simulink model "Suspension7DoF_GDP_Final"  (R2025a)
settings: Solver=ode4  StartTime=0.0  StopTime=209.85  FixedStep=0.001  RelTol=1e-3
undefined symbols (not defined in the file): A, Bl, Cl_table, cmax_f, cmax_r, cmax_roll_f, cmax_roll_r, cmin_f, cmin_r, cmin_roll_f, cmin_roll_r, cog_z, cog_z_us, CoP_x_table, CoP_y, g, Ixx, Iyy, k_roll_f, k_roll_r, kf, kr, kt, Lf, Lr, m_s, m_s_a, m_s_b, m_us, rake_breaks, RC_F_z, RC_R_z, RH_breaks, rho, roll_centre_z, Tr
libraries: simulink x2
settings Model: Creator=alexw  LastModifiedBy=alexw

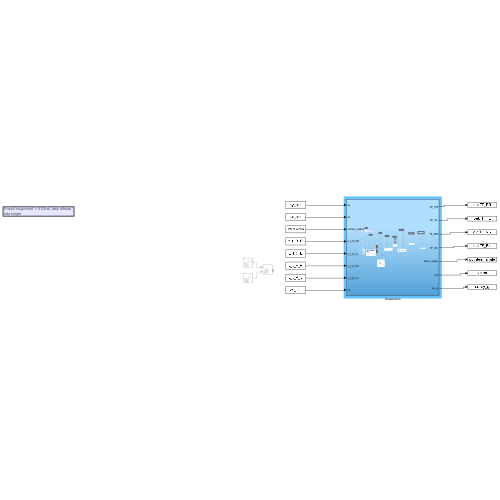
[thumbnail: Simulink's stored preview of the top-level diagram]
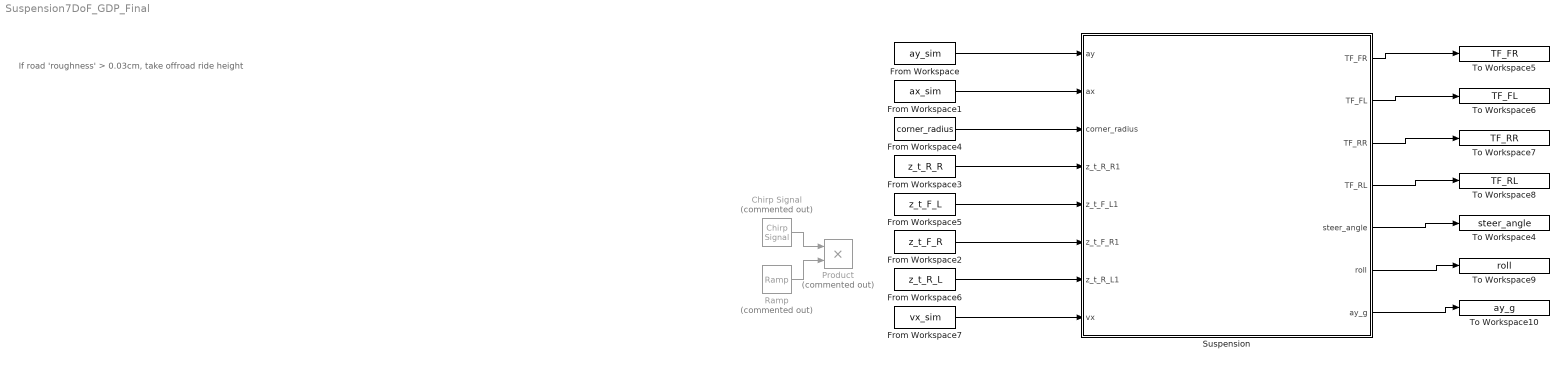
== system Suspension7DoF_GDP_Final ==
  note: If road 'roughness' > 0.03cm, take offroad
      | ride height
  Chirp Signal : simulink/Sources/Chirp Signal  Commented=on  f1=0.1  T=100  f2=20
  From Workspace : FromWorkspace  VariableName=ay_sim
  From Workspace1 : FromWorkspace  VariableName=ax_sim
  From Workspace2 : FromWorkspace  VariableName=z_t_F_R
  From Workspace3 : FromWorkspace  VariableName=z_t_R_R
  From Workspace4 : FromWorkspace  VariableName=corner_radius
  From Workspace5 : FromWorkspace  VariableName=z_t_F_L
  From Workspace6 : FromWorkspace  VariableName=z_t_R_L
  From Workspace7 : FromWorkspace  VariableName=vx_sim
  Product : Product  Commented=on
  Ramp : simulink/Sources/Ramp  Commented=on  slope=-0.0001  start=0  InitialOutput=0.01
  Suspension : Subsystem
  To Workspace10 : ToWorkspace  VariableName=ay_g  SaveFormat=Timeseries  SampleTime=-1
  To Workspace4 : ToWorkspace  VariableName=steer_angle  SaveFormat=Timeseries  SampleTime=-1
  To Workspace5 : ToWorkspace  VariableName=TF_FR  SaveFormat=Timeseries  SampleTime=-1
  To Workspace6 : ToWorkspace  VariableName=TF_FL  SaveFormat=Timeseries  SampleTime=-1
  To Workspace7 : ToWorkspace  VariableName=TF_RR  SaveFormat=Timeseries  SampleTime=-1
  To Workspace8 : ToWorkspace  VariableName=TF_RL  SaveFormat=Timeseries  SampleTime=-1
  To Workspace9 : ToWorkspace  VariableName=roll  SaveFormat=Timeseries  SampleTime=-1
  wires:
  Chirp Signal/1 -> Product/1
  Ramp/1 -> Product/2
  From Workspace/1 -> Suspension/1(ay)
  From Workspace1/1 -> Suspension/2(ax)
  From Workspace3/1 -> Suspension/4(z_t_R_R1)
  Suspension/1(TF_FR) -> To Workspace5/1
  Suspension/2(TF_FL) -> To Workspace6/1
  Suspension/3(TF_RR) -> To Workspace7/1
  Suspension/4(TF_RL) -> To Workspace8/1
  Suspension/5(steer_angle) -> To Workspace4/1
  From Workspace4/1 -> Suspension/3(corner_radius)
  From Workspace5/1 -> Suspension/5(z_t_F_L1)
  Suspension/6(roll) -> To Workspace9/1
  Suspension/7(ay_g) -> To Workspace10/1
  From Workspace7/1 -> Suspension/8(vx)
  From Workspace6/1 -> Suspension/7(z_t_R_L1)
  From Workspace2/1 -> Suspension/6(z_t_F_R1)

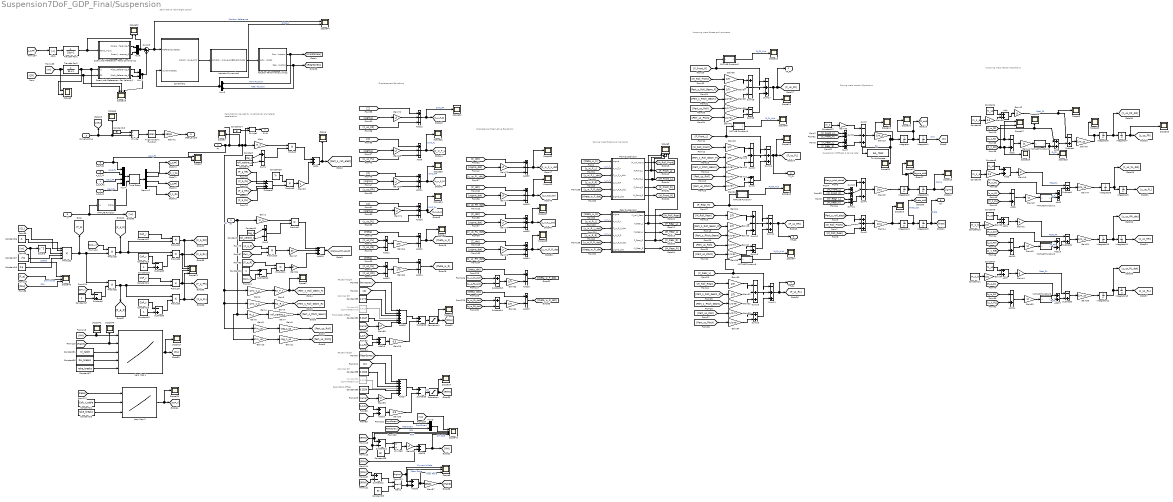
== system Suspension7DoF_GDP_Final/Suspension ==
  note: Suspension Stiffness = spring rate:
  note: Unsprung mass Newton Equations
  note: Sprung mass newton Equations
  note: Unsprung mass forces and moments
  note: Sprung mass forces and moments
  note: Displacement Derivative Equations
  note: Displacement Equations
  note: Perturbations caused by
      | longitudinal and lateral acceleration
  note: Front Static Offset
  note: Rear Static Offset
  note: Raised height
  note: Raised height
  note: Nominal RH
  note: Nominal RH
  note: Semi-Active ride height control
  ay : Inport
  ax : Inport  Port=2
  corner_radius : Inport  Port=3
  z_t_R_R1 : Inport  Port=4
  z_t_F_L1 : Inport  Port=5
  z_t_F_R1 : Inport  Port=6
  z_t_R_L1 : Inport  Port=7
  vx : Inport  Port=8
  Abs1 : Abs  SaturateOnIntegerOverflow=off
  Actuator Dynamics1 : Subsystem
  Actuator Performance Limits1 : Subsystem
  Add{,1,3..5,7,9,13,17,19..20,28,30} (13 alike) : Sum
  Add{2,6,10,14} (4 alike) : Sum  Inputs=-+
  Add{11,16,34..35} (4 alike) : Sum  Inputs=++-
  Add{8,12,15,33} (4 alike) : Sum  Inputs=+--
  Add18 : Sum  Inputs=+++
  Add{21..25,29} (6 alike) : Sum  Inputs=+-
  Add26 : Sum  Inputs=++++++
  Add27 : Sum  Inputs=++++++
  Aero Map 1 : Lookup_n-D  LookupTableObject=h  BreakpointsForDimension1Source=Input port  BreakpointsForDimension1=[0:0.01:0.2]  BreakpointsForDimension2Source=Input port  BreakpointsForDimension2=[-10:10]  TableSource=Input port  InternalRulePriority=Speed  RndMeth=Simplest
      settings: InputPortMap=u0,u1,p221,p5,p7
  Aero Map 2 : Lookup_n-D  NumberOfTableDimensions=1  BreakpointsForDimension1Source=Input port  BreakpointsForDimension1=[-5:5]  TableSource=Input port  Table=tanh([-5:5])  InternalRulePriority=Speed  RndMeth=Simplest
      settings: InputPortMap=u0,p221,p5
  Atan2 : Trigonometry  Operator=atan2
  Constant : Constant  Value=cog_z
  Constant1 : Constant  Value=roll_centre_z
  Constant10 : Constant  Value=m_s_b
  Constant11 : Constant  Value=m_s_b
  Constant12 : Constant  Value=m_s
  Constant13 : Constant  Value=Bl
  Constant14 : Constant  Value=g
  Constant15 : Constant  Commented=on  Value=0.025
  Constant16 : Constant  Value=0.5
  Constant{17..20} (4 alike) : Constant
  Constant2 : Constant  Value=cog_z
  Constant21 : Constant  Value=CoP_x_table  VectorParams1D=off
  Constant{22..25} (4 alike) : Constant  Value=CoP_y
  Constant26 : Constant  Value=A
  Constant27 : Constant  Value=rho
  Constant28 : Constant  Value=Tr
  Constant29 : Constant  Value=rake_breaks  VectorParams1D=off
  Constant3 : Constant  Value=roll_centre_z
  Constant30 : Constant  Value=0.1154
  Constant31 : Constant  Value=Cl_table  VectorParams1D=off
  Constant32 : Constant  Value=0.1447
  Constant33 : Constant  Value=Bl
  Constant34 : Constant  Commented=on  Value=0.025
  Constant35 : Constant  Value=0.1043
  Constant36 : Constant  Value=RH_breaks  VectorParams1D=off
  Constant37 : Constant  Value=rake_breaks  VectorParams1D=off
  Constant38 : Constant  Value=Bl
  Constant39 : Constant  Value=0.075
  Constant{4..7} (4 alike) : Constant  Value=m_us
  Constant8 : Constant  Value=m_s_a
  Constant9 : Constant  Value=m_s_a
  Controller1 : Subsystem
  Demux1 : Demux
  Divide : Product  Inputs=*/
  Divide1 : Product  Inputs=*/
  Divide3 : Product  Inputs=*/
  Front Suspension : Subsystem  mask(half-car suspension){kf=kf, kthetaf=-k_roll_f, cmin_f=cmin_f, cmax_f=cmax_f, cmin_thetaf=cmin_roll_f, cmax_thetaf=cmax_roll_f, Lr=Lr}
      mask prompts: kf "Suspension Stiffness"; kthetaf "Roll Stiffness:"; cmin_f "Minmum Suspension Damping:"; cmax_f "Maximum Suspension Damping:"; cmin_thetaf "Minimum Roll Damping:"; cmax_thetaf "Maximum Roll Damping:"; Lr "Moment Arm:"
      mask help:
      | Half-Car Suspension
      | The spring and damping rates for an individual wheel are entered below.  Their combined effect as applied to two wheels at the specified distance from the center of mass is computed.  The distance should be specified as positive if the subsystem is oriented such that increasing z corresponds to increasing theta, negative otherwise.
      mask Help: See "Using Simulink and Stateflow in Automotive Applications" for a mathematical derivation of the subsystem operation.  Contact your MathWorks distributor to obtain a copy.
      mask Display: plot(-1, 0, 13, 12, [1 12], [11 11], [1 5], [2 2], [1 2], [4.5 5], [2 0], [5 6], [0 2], [6 7], [2 0], [7 8], [0 1], [8 8.5], [1 1], [8.5 11], [1 1], [2 4.5], [5 5], [2 5], [4 6], [5 5], [4 4], [5 8], [6 6], [5 8], [4 6], [6.5 6.5], [5 5], [6.5 11], [0 1], [1 2], [2 3], [1 2], [4 5], [1 2])
  Gain : Gain  Gain=m_s
  Gain1 : Gain  Gain=m_s
  Gain10 : Gain  Gain=4*m_us
  Gain11 : Gain  Gain=cog_z_us
  Gain{12,16,42,44,46} (5 alike) : Gain  Gain=g
  Gain13 : Gain  Gain=1/m_s
  Gain14 : Gain  Gain=1/Ixx
  Gain15 : Gain  Gain=1/Iyy
  Gain17 : Gain  Gain=Bl
  Gain{18..19,24..25,30..31,36..37,60..62,64} (12 alike) : Gain  Gain=1/Tr
  Gain2 : Gain  Gain=-1*m_s_a
  Gain{20,22,26,28,32,34,38,40} (8 alike) : Gain  Gain=1/(2*Bl)
  Gain{21,27,33,39} (4 alike) : Gain  Gain=1/(2*Tr)
  Gain23 : Gain
  Gain{29,35,48,50,52,54} (6 alike) : Gain  Gain=0.5
  Gain3 : Gain  Gain=RC_F_z
  Gain4 : Gain  Gain=-1*m_s_b
  Gain{41,45,49,53} (4 alike) : Gain  Gain=kt
  Gain{43,47,51,55} (4 alike) : Gain  Gain=1/m_us
  Gain5 : Gain  Gain=RC_R_z
  Gain56 : Gain  Gain=Bl
  Gain57 : Gain  Gain=180/pi
  Gain{58,63,68,70,73..74} (6 alike) : Gain  Gain=Lf
  Gain59 : Gain  Gain=-Lr
  Gain6 : Gain  Gain=m_s
  Gain{69,71,75..76} (4 alike) : Gain  Gain=Lr
  Gain7 : Gain  Gain=roll_centre_z
  Gain72 : Gain  Gain=180/pi
  Gain8 : Gain  Gain=4*m_us
  Gain9 : Gain  Gain=cog_z_us
  Integrator{,1..13} (14 alike) : Integrator
  MATLAB Function : MATLAB Function  TreatAsAtomicUnit=on
  MATLAB Function1 : MATLAB Function  TreatAsAtomicUnit=on
  MATLAB Function2 : MATLAB Function  TreatAsAtomicUnit=on
  MATLAB Function3 : MATLAB Function  TreatAsAtomicUnit=on
  MATLAB Function4 : MATLAB Function  TreatAsAtomicUnit=on
  MATLAB Function5 : MATLAB Function  TreatAsAtomicUnit=on
  MATLAB Function6 : MATLAB Function  TreatAsAtomicUnit=on
  MATLAB Function7 : MATLAB Function  TreatAsAtomicUnit=on
  MATLAB Function8 : MATLAB Function  TreatAsAtomicUnit=on
  Mux{3,5..7} (4 alike) : Mux  Inputs=2
  Mux4 : Mux
  Product{,1,3..11} (11 alike) : Product
  Product2 : Product  Inputs=5
  Rear Suspension : Subsystem  mask(half-car suspension){kr=kr, kthetar=-k_roll_r, cmin_r=cmin_r, cmax_r=cmax_r, cmin_thetar=cmin_roll_r, cmax_thetar=cmax_roll_r, Lr=Lr}
      mask prompts: kr "Suspension Stiffness:"; kthetar "Roll Stiffness:"; cmin_r "Minimum Suspension Damping:"; cmax_r "Maximum Suspension Damping:"; cmin_thetar "Minimum Roll Damping:"; cmax_thetar "Maximum Roll Damping:"; Lr "Moment Arm:"
      mask help:
      | Half-Car Suspension
      | The spring and damping rates for an individual wheel are entered below.  Their combined effect as applied to two wheels at the specified distance from the center of mass is computed.  The distance should be specified as positive if the subsystem is oriented such that increasing z corresponds to increasing theta, negative otherwise.
      mask Help: See "Using Simulink and Stateflow in Automotive Applications" for a mathematical derivation of the subsystem operation.  Contact your MathWorks distributor to obtain a copy.
      mask Display: plot(-1, 0, 13, 12, [1 12], [11 11], [1 5], [2 2], [1 2], [4.5 5], [2 0], [5 6], [0 2], [6 7], [2 0], [7 8], [0 1], [8 8.5], [1 1], [8.5 11], [1 1], [2 4.5], [5 5], [2 5], [4 6], [5 5], [4 4], [5 8], [6 6], [5 8], [4 6], [6.5 6.5], [5 5], [6.5 11], [0 1], [1 2], [2 3], [1 2], [4 5], [1 2])
  Saturation : Saturate  LowerLimit=0
  Saturation1 : Saturate  LowerLimit=0
  Scope{,1..4,6,10..15,17..20,23..26,28..39,42..43,45..47} (37 alike) : Scope
      Scope settings: DataLoggingVariableName=ScopeData28
      Scope1 settings: ActiveDisplayYMinimum=-15.845612610428327  ActiveDisplayYMaximum=15.435881700857845  DataLoggingVariableName=ScopeData13
      Scope10 settings: ActiveDisplayYMinimum=-1  ActiveDisplayYMaximum=1  DataLoggingVariableName=ScopeData14
      Scope11 settings: ActiveDisplayYMinimum=-1  ActiveDisplayYMaximum=1  DataLoggingVariableName=ScopeData15
      Scope12 settings: ActiveDisplayYMinimum=-1  ActiveDisplayYMaximum=1  DataLoggingVariableName=ScopeData16
      Scope13 settings: ActiveDisplayYMinimum=-0.11164438440318229  ActiveDisplayYMaximum=0.015517013432769977  DataLoggingVariableName=ScopeData17
      Scope14 settings: ActiveDisplayYMinimum=-1  ActiveDisplayYMaximum=1  DataLoggingVariableName=ScopeData18
      Scope15 settings: DataLoggingVariableName=ScopeData19
      Scope17 settings: ActiveDisplayYMinimum=-1.4006676134136735  ActiveDisplayYMaximum=0.60935482779584749  DataLoggingVariableName=ScopeData35
      Scope18 settings: DataLoggingVariableName=ScopeData22
      Scope19 settings: ActiveDisplayYMinimum=-1  ActiveDisplayYMaximum=1  DataLoggingVariableName=ScopeData23
      Scope2 settings: ActiveDisplayYMinimum=-1  ActiveDisplayYMaximum=1  DataLoggingVariableName=ScopeData6
      Scope20 settings: ActiveDisplayYMinimum=-1  ActiveDisplayYMaximum=1  DataLoggingVariableName=ScopeData24
      Scope23 settings: ActiveDisplayYMinimum=-1  ActiveDisplayYMaximum=1  DataLoggingVariableName=ScopeData36
      Scope24 settings: ActiveDisplayYMinimum=-1  ActiveDisplayYMaximum=1  DataLoggingVariableName=ScopeData37
      Scope25 settings: ActiveDisplayYMinimum=-2095.00512229594  ActiveDisplayYMaximum=18855.046100663465  DataLoggingVariableName=ScopeData29
      Scope26 settings: ActiveDisplayYMinimum=-0.15055367778646628  ActiveDisplayYMaximum=0.064777386245955387  DataLoggingVariableName=ScopeData30
      Scope28 settings: ActiveDisplayYMinimum=-0.00037040753132380039  ActiveDisplayYMaximum=0.0017989620179888006  DataLoggingVariableName=ScopeData32
      Scope29 settings: ActiveDisplayYMinimum=-14729.679405263418  ActiveDisplayYMaximum=5136.5247908965184  DataLoggingVariableName=ScopeData33
      Scope3 settings: ActiveDisplayYMinimum=-1  ActiveDisplayYMaximum=1  DataLoggingVariableName=ScopeData7
      Scope30 settings: ActiveDisplayYMinimum=-1  ActiveDisplayYMaximum=1  DataLoggingVariableName=ScopeData34
      Scope31 settings: ActiveDisplayYMinimum=-0.35226875587213935  ActiveDisplayYMaximum=0.075007941544787432  DataLoggingVariableName=ScopeData6
      Scope32 settings: ActiveDisplayYMinimum=-0.26331111069166768  ActiveDisplayYMaximum=0.0678002738486741  DataLoggingVariableName=ScopeData29
      Scope33 settings: ActiveDisplayYMinimum=-0.28108589618879348  ActiveDisplayYMaximum=0.05450271554919274  DataLoggingVariableName=ScopeData4
      Scope34 settings: ActiveDisplayYMinimum=-0.024162682451583074  ActiveDisplayYMaximum=0.024369090839316668  DataLoggingVariableName=ScopeData5
      Scope35 settings: ActiveDisplayYMinimum=-1.8920079045633775  ActiveDisplayYMaximum=1.5269548555882952
      Scope36 settings: ActiveDisplayYMinimum=-1.8920079045633775  ActiveDisplayYMaximum=1.5269548555882952
      Scope37 settings: ActiveDisplayYMinimum=-2.8014124962622828  ActiveDisplayYMaximum=2.3840420433740279  DataLoggingVariableName=ScopeData2
      Scope38 settings: ActiveDisplayYMinimum=-2.8014124962622828  ActiveDisplayYMaximum=2.3840420433740279  DataLoggingVariableName=ScopeData3
      Scope39 settings: ActiveDisplayYMinimum=-1  ActiveDisplayYMaximum=1  DataLoggingVariableName=ScopeData38
      Scope4 settings: ActiveDisplayYMinimum=-1  ActiveDisplayYMaximum=1  DataLoggingVariableName=ScopeData8
      Scope42 settings: ActiveDisplayYMinimum=-1  ActiveDisplayYMaximum=1  DataLoggingVariableName=ScopeData41
      Scope43 settings: ActiveDisplayYMinimum=-9.022413114497672  ActiveDisplayYMaximum=5.2150908469293062  DataLoggingVariableName=ScopeData42
      Scope45 settings: DataLoggingVariableName=ScopeData20
      Scope46 settings: DataLoggingVariableName=ScopeData45
      Scope47 settings: DataLoggingVariableName=ScopeData46
      Scope6 settings: ActiveDisplayYMinimum=-20.40704420043474  ActiveDisplayYMaximum=1207.4194628810842  DataLoggingVariableName=ScopeData10
  Scope16 : Scope  NumInputPorts=3
      settings: ActiveDisplayString=3  ActiveDisplayYMinimum=-0.012499999999999997  ActiveDisplayYMaximum=0.1125  DataLoggingVariableName=ScopeData27
  Scope21 : Scope  NumInputPorts=4
      settings: ActiveDisplayYMinimum=-1  ActiveDisplayYMaximum=1  DataLoggingVariableName=ScopeData26
  Scope{7..8,22,27,44} (5 alike) : Scope  NumInputPorts=2
      Scope22 settings: ActiveDisplayYMinimum=-0.0093749999999999979  ActiveDisplayYMaximum=0.084374999999999992  DataLoggingVariableName=ScopeData43
      Scope27 settings: ActiveDisplayYMinimum=-1  ActiveDisplayYMaximum=1  DataLoggingVariableName=ScopeData31
      Scope44 settings: ActiveDisplayYMinimum=-0.012499999999999997  ActiveDisplayYMaximum=0.1125  DataLoggingVariableName=ScopeData44
      Scope7 settings: ActiveDisplayYMinimum=-11.512910069370855  ActiveDisplayYMaximum=11.657951350029352  DataLoggingVariableName=ScopeData11
      Scope8 settings: ActiveDisplayYMinimum=-1  ActiveDisplayYMaximum=1
  Scope40 : Scope  NumInputPorts=3
      settings: ActiveDisplayYMinimum=-1  ActiveDisplayYMaximum=1  DataLoggingVariableName=ScopeData39
  Scope41 : Scope  NumInputPorts=5
      settings: ActiveDisplayYMinimum=-6.374509016200431  ActiveDisplayYMaximum=57.4705811458039  DataLoggingVariableName=ScopeData40
  Scope5 : Scope  NumInputPorts=3
      settings: ActiveDisplayYMinimum=-1  ActiveDisplayYMaximum=1  DataLoggingVariableName=ScopeData9
  Scope9 : Scope  NumInputPorts=4
      settings: ActiveDisplayYMinimum=-1  ActiveDisplayYMaximum=1  DataLoggingVariableName=ScopeData25
  Screw jack Reference - Car Velocity1 : MATLAB Function  TreatAsAtomicUnit=on
  Screw jack Reference - Road Conditions1 : MATLAB Function  TreatAsAtomicUnit=on
  Square : Math  Operator=square
  Subtract{,1..6} (7 alike) : Sum  Inputs=-+
  Subtract{8..14} (7 alike) : Sum  Inputs=+-
  Subtract7 : Sum  Inputs=+-+-
  Sum1 : Sum  Inputs=|+-
  Sum{10..11,14..15,17} (5 alike) : Sum  Inputs=|-++
  Sum12 : Sum  Inputs=|+-+
  Sum13 : Sum  Inputs=|-+
  Sum16 : Sum  Inputs=|++
  Sum18 : Sum  Inputs=|+--
  Sum19 : Sum  Inputs=|--
  Sum2 : Sum  Inputs=|+-
  Sum{5,7,20..21} (4 alike) : Sum
  Sum23 : Sum  Inputs=|++
  Sum3 : Sum  Inputs=-++
  Sum4 : Sum  Inputs=|+-+
  Sum6 : Sum  Inputs=|+++
  Sum8 : Sum  Inputs=|-+-
  Sum9 : Sum  Inputs=|+-
  Time Delay : VariableTransportDelay  MaximumDelay=10  MaximumPoints=10240  FixedBuffer=on  ZeroDelay=on
  To Workspace : ToWorkspace  VariableName=BA_7DoF  SampleTime=-1
      settings: Save2DSignal=2-D array (concatenate along first dimension)
  Transfer Fcn1 : TransferFcn  Denominator=[10 1]
  Transfer Fcn2 : TransferFcn  Denominator=[3 1]
  Trigonometric Function : Trigonometry  Operator=atan
  TF_FR : Outport
  TF_FL : Outport  Port=2
  TF_RR : Outport  Port=3
  TF_RL : Outport  Port=4
  steer_angle : Outport  Port=5
  roll : Outport  Port=6
  ay_g : Outport  Port=7
  wires:
  Gain/1 -> Product/1
  Constant1/1 -> Sum1/2
  Constant/1 -> Sum1/1
  Sum1/1 -> Product/2
  Constant2/1 -> Sum2/1
  Constant3/1 -> Sum2/2
  Gain1/1 -> Product1/1
  ax/1 -> Gain1/1, Gain10/1, Gain6/1
  Sum2/1 -> Product1/2
  Gain2/1 -> Gain3/1
  Gain4/1 -> Gain5/1
  Gain3/1 -> Scope2/1, [Pert_s_Roll_Geom_F]
  Gain5/1 -> [Pert_s_Roll_Geom_R]
  Gain6/1 -> Gain7/1
  Gain7/1 -> [Pert_s_Pitch_Geom]
  Gain8/1 -> Gain9/1
  Gain10/1 -> Gain11/1
  Gain9/1 -> [Pert_us_Roll]
  Gain11/1 -> [Pert_us_Pitch]
  Sum3/1 -> Gain13/1
  Gain13/1 -> To Workspace/1, Scope30/1, Scope11/1, Integrator/1  "BA"
  Integrator/1 -> Scope10/1, [Z_dot], Integrator1/1
  Integrator2/1 -> Scope12/1, [sigma_dot], Integrator3/1
  Gain15/1 -> Integrator2/1
  Sum4/1 -> Gain15/1
  [Pert_s_pitch_elast] -> Sum4/1
  [Pert_s_roll_elast] -> Sum6/1
  Integrator5/1 -> roll/1, [theta]  "theta"
  Sum6/1 -> Gain14/1
  [M_Roll_Rear] -> Sum6/3
  [M_Roll_Front] -> Sum6/2
  Gain14/1 -> Scope19/1, Integrator4/1
  Sum8/1 -> Sum10/2
  Sum9/1 -> Sum10/3
  Sum10/1 -> TF_FL/1, Scope18/1, [F_us_FL]
  [M_Roll_Front] -> Gain18/1
  Gain18/1 -> Sum8/1
  [Pert_s_Roll_Geom_F] -> Gain19/1
  Gain19/1 -> Sum8/2
  [Pert_s_Pitch_Geom] -> Gain20/1
  Gain20/1 -> Sum8/3
  [Pert_us_Roll] -> Gain21/1
  Gain21/1 -> Sum9/1
  [Pert_us_Pitch] -> Gain22/1
  Gain22/1 -> Sum9/2
  Gain27/1 -> Sum13/1
  Gain28/1 -> Sum13/2
  [Pert_us_Roll] -> Gain27/1
  Gain26/1 -> Sum12/3
  [Pert_s_Pitch_Geom] -> Gain26/1
  Gain24/1 -> Sum12/1
  [Pert_s_Roll_Geom_R] -> Gain25/1
  Gain25/1 -> Sum12/2
  Sum11/1 -> TF_RR/1, [F_us_RR]
  Sum12/1 -> Sum11/2
  [Pert_us_Pitch] -> Gain28/1
  Sum13/1 -> Sum11/3
  [M_Roll_Rear] -> Gain24/1
  Gain33/1 -> Sum16/1
  Gain34/1 -> Sum16/2
  [Pert_us_Roll] -> Gain33/1
  Gain32/1 -> Sum15/3
  [Pert_s_Pitch_Geom] -> Gain32/1
  Gain30/1 -> Sum15/1
  [Pert_s_Roll_Geom_R] -> Gain31/1
  Gain31/1 -> Sum15/2
  Sum14/1 -> TF_RL/1, [F_us_RL]
  Sum15/1 -> Sum14/2
  [Pert_us_Pitch] -> Gain34/1
  Sum16/1 -> Sum14/3
  [M_Roll_Rear] -> Gain30/1
  Gain39/1 -> Sum19/1
  [F_Front_R] -> MATLAB Function5/1(u), Sum17/1
  Gain40/1 -> Sum19/2
  [Pert_us_Roll] -> Gain39/1
  Gain38/1 -> Sum18/3
  [Pert_s_Pitch_Geom] -> Gain38/1
  Gain36/1 -> Sum18/1
  [Pert_s_Roll_Geom_F] -> Gain37/1
  Gain37/1 -> Sum18/2
  Sum17/1 -> Scope14/1, TF_FR/1, [F_us_FR]
  Sum18/1 -> Sum17/2
  [Pert_us_Pitch] -> Gain40/1
  Sum19/1 -> Sum17/3
  [M_Roll_Front] -> Gain36/1
  [z_us_FR] -> Scope27/1, Add2/1
  [z_t_FR] -> Scope27/2, Add2/2, Scope28/1
  Add2/1 -> Gain41/1
  Add5/1 -> Subtract/2
  Integrator7/1 -> Scope26/1, [z_us_FR]
  Gain43/1 -> Scope20/1, Integrator6/1
  Integrator6/1 -> Integrator7/1, [z_us_FR_dot]
  [z_t_FL] -> Add6/2
  Gain47/1 -> Integrator8/1
  Add9/1 -> Subtract1/2
  Add6/1 -> Gain45/1
  [z_us_FL] -> Add6/1
  Integrator8/1 -> Integrator9/1, [z_us_FL_dot]
  Integrator9/1 -> [z_us_FL]
  [z_t_RR] -> Add10/2
  Gain51/1 -> Integrator10/1
  Add13/1 -> Subtract2/2
  Add10/1 -> Gain49/1
  [z_us_RR] -> Add10/1
  Integrator10/1 -> Integrator11/1, [z_us_RR_dot]
  Integrator11/1 -> [z_us_RR]
  [z_t_RL] -> Add14/2
  Gain55/1 -> Integrator12/1
  Add17/1 -> Subtract3/2
  Add14/1 -> Gain53/1
  [z_us_RL] -> Add14/1
  Integrator12/1 -> Integrator13/1, [z_us_RL_dot]
  Integrator13/1 -> [z_us_RL]
  Add21/1 -> Gain61/1
  [z_us_FL] -> Add21/1
  [theta] -> Add22/1
  Add22/1 -> Scope4/1, [theta_w_F]
  [z_us_FR] -> Add21/2
  Gain61/1 -> Add22/2
  Add24/1 -> [theta_w_R]
  [z_us_RR] -> Add23/2
  Add23/1 -> Gain60/1
  [theta] -> Add24/1
  [z_us_RL] -> Add23/1
  Gain60/1 -> Add24/2
  [F_us_FR] -> Add5/1, Scope29/1
  [F_us_FL] -> Add9/1
  Gain45/1 -> MATLAB Function1/1(u)
  [F_us_RR] -> Add13/1
  Gain49/1 -> MATLAB Function2/1(u)
  [F_us_RL] -> Add17/1
  Gain53/1 -> MATLAB Function3/1(u)
  MATLAB Function1/1(y) -> Add9/2  "Ft_FL"
  MATLAB Function2/1(y) -> Add13/2  "Ft_RR"
  MATLAB Function3/1(y) -> Add17/2  "Ft_RL"
  Gain41/1 -> MATLAB Function4/1(u)
  MATLAB Function4/1(y) -> Add5/2, Scope25/1  "Ft_FR"
  Constant4/1 -> Add/1
  Gain16/1 -> Subtract1/1  "Fstat_FL"
  Gain42/1 -> Subtract2/1  "Fstat_RR"
  Gain44/1 -> Subtract3/1  "Fstat_RL"
  Add/1 -> Gain12/1
  Constant8/1 -> Gain48/1
  Constant5/1 -> Add3/1
  Add3/1 -> Gain16/1
  Constant6/1 -> Add4/1
  Gain52/1 -> Add4/2
  Add4/1 -> Gain42/1
  Constant7/1 -> Add7/1
  Gain54/1 -> Add7/2
  Add7/1 -> Gain44/1
  Constant12/1 -> Gain46/1
  Gain46/1 -> Sum3/1
  Gain48/1 -> Add/2
  Constant9/1 -> Gain50/1
  Gain50/1 -> Add3/2
  Constant10/1 -> Gain52/1
  Constant11/1 -> Gain54/1
  Subtract/1 -> Gain43/1
  Gain12/1 -> Scope3/1, Subtract/1  "Fstat_FR"
  Subtract1/1 -> Gain47/1
  Subtract2/1 -> Gain51/1
  Subtract3/1 -> Gain55/1
  Add12/1 -> [z_w_F_R], Scope31/1  "SWS_FR"
  [sigma] -> Gain68/1
  Add11/1 -> Scope33/1, [z_w_R_R]  "SWS_RR"
  [sigma] -> Gain70/1
  [z_us_FR] -> Add12/3
  [z_us_FL] -> Add8/3
  [z_us_RL] -> Add16/3
  Add8/1 -> [z_w_F_L], Scope32/1  "SWS_FL"
  [sigma] -> Gain69/1
  Gain69/1 -> Add11/2
  Gain68/1 -> Add8/2
  [sigma] -> Gain71/1
  Gain70/1 -> Add12/2
  Gain71/1 -> Add16/2
  [z_us_RR] -> Add11/3
  Add16/1 -> Scope34/1, [z_w_R_L]  "SWS_RL"
  corner_radius/1 -> [CR], Scope6/1, Divide/2
  Trigonometric Function/1 -> Gain72/1
  Gain72/1 -> steer_angle/1
  Divide/1 -> Trigonometric Function/1
  Constant13/1 -> Divide/1
  [sigma_dot] -> Gain75/1
  Add33/1 -> Scope35/1, [z_w_F_L_dot]
  Add35/1 -> Scope37/1, [z_w_R_L_dot]
  Gain75/1 -> Add35/2
  [Z_dot] -> Add35/1
  Gain73/1 -> Add33/2
  [sigma_dot] -> Gain73/1
  [Z_dot] -> Add33/1
  [z_us_FL_dot] -> Add33/3
  [sigma_dot] -> Gain74/1
  Add15/1 -> Scope36/1, [z_w_F_R_dot]
  Gain74/1 -> Add15/2
  [z_us_FR_dot] -> Add15/3
  [Z_dot] -> Add15/1
  [z_us_RL_dot] -> Add35/3
  Add34/1 -> Scope38/1, [z_w_R_R_dot]
  [sigma_dot] -> Gain76/1
  [Z_dot] -> Add34/1
  Gain76/1 -> Add34/2
  [z_us_RR_dot] -> Add34/3
  [F_Front_L] -> Sum5/1
  [F_Front_R] -> Sum5/2
  Sum5/1 -> Sum3/2
  [F_Rear_L] -> Sum7/1
  [F_Rear_R] -> Sum7/2
  Sum7/1 -> Sum3/3
  [M_Rear_R] -> Sum21/2
  [M_Rear_L] -> Sum21/1
  [M_Front_L] -> Sum20/1
  [M_Front_R] -> Sum20/2
  Sum20/1 -> Sum4/2
  Sum21/1 -> Sum4/3
  Divide1/1 -> ay_g/1
  Constant14/1 -> Divide1/2
  [Z] -> Add12/1
  [Z] -> Add8/1
  [vx] -> Scope40/1, Square/1  "Speed"
  Constant27/1 -> Product2/4
  Constant16/1 -> Product2/5
  Square/1 -> Product2/3
  Product2/1 -> Product5/1, Product3/2, [F_a]
  Product3/1 -> [F_a_R], Product4/2, Product6/1
  Constant22/1 -> Product4/1
  Product4/1 -> Scope21/1, [F_a_RR]
  Constant17/1 -> Subtract4/2
  [CoP_x] -> Subtract4/1
  Subtract4/1 -> Product5/2
  Constant18/1 -> Subtract5/2
  Subtract5/1 -> Product6/2
  Product6/1 -> Scope21/2, [F_a_RL]
  Product7/1 -> [F_a_FR], Scope21/3
  Constant24/1 -> Product7/1
  Product5/1 -> Product8/1, Product7/2, [F_a_F]
  Constant19/1 -> Subtract6/2
  Constant25/1 -> Subtract6/1
  Subtract6/1 -> Product8/2
  [CoP_x] -> Product3/1
  Constant23/1 -> Subtract5/1
  Product8/1 -> [F_a_FL], Scope21/4
  [F_a_FR] -> Subtract7/1
  Constant28/1 -> Product9/1
  Subtract7/1 -> Product9/2
  Product9/1 -> Gain23/1
  [F_a_FL] -> Subtract7/2
  [F_a_RR] -> Subtract7/3
  [F_a_RL] -> Subtract7/4
  Product/1 -> Add1/1
  Gain23/1 -> Add1/2
  Add1/1 -> [Pert_s_roll_elast], Scope/1
  Product1/1 -> Add18/1
  Gain17/1 -> Add18/2
  Gain56/1 -> Add18/3
  Add18/1 -> [Pert_s_pitch_elast]
  [z_t_FL] -> Add19/1
  [z_t_FR] -> Add19/2
  Add19/1 -> Gain29/1
  Add20/1 -> Gain35/1
  [z_t_RR] -> Add20/2
  [z_t_RL] -> Add20/1
  [Z] -> Add26/2
  Constant32/1 -> Add26/5
  Subtract9/1 -> Saturation/1  "RRH"
  Saturation/1 -> Scope24/1, [RRH]
  [sigma] -> Gain58/1
  [sigma] -> Gain59/1
  Gain58/1 -> Add26/6
  [Z] -> Add27/2
  Constant30/1 -> Add27/5
  Gain59/1 -> Add27/6
  Add26/1 -> Subtract8/1
  Gain29/1 -> Subtract8/2
  Subtract8/1 -> Saturation1/1
  Saturation1/1 -> Scope23/1, [FRH]
  Gain35/1 -> Subtract9/2
  Add27/1 -> Subtract9/1
  Divide3/1 -> Gain63/1
  [FRH] -> Subtract11/2, Scope41/3  "FRH"
  [RRH] -> Subtract11/1, Scope41/4  "RRH"
  [FRH] -> Add28/2
  Constant38/1 -> Divide3/2
  Gain63/1 -> Add28/1
  Subtract11/1 -> Divide3/1
  Add28/1 -> [RH], Scope41/5  "RH COG"
  [Rake] -> Aero Map 2/1
  Constant21/1 -> Aero Map 2/2
  Constant29/1 -> Aero Map 2/3
  Constant31/1 -> Aero Map 1/3
  [Rake] -> Aero Map 1/2, Scope43/1
  Constant37/1 -> Aero Map 1/5
  Aero Map 2/1 -> Scope39/1, [CoP_x]
  Constant36/1 -> Aero Map 1/4
  [RH] -> Scope42/1, Aero Map 1/1
  Aero Map 1/1 -> Scope17/1, [CL]
  [CL] -> Product2/1
  Product10/1 -> Gain17/1
  [F_a_F] -> Product10/1
  [CoP_x] -> Product10/2
  Constant20/1 -> Subtract10/1
  [CoP_x] -> Subtract10/2
  Product11/1 -> Gain56/1
  [F_a_R] -> Product11/1
  Subtract10/1 -> Product11/2
  [F_a] -> Scope40/2  "Downforce"
  Constant26/1 -> Product2/2
  [Z] -> Add11/1
  [Z] -> Add16/1
  Integrator1/1 -> [Z]  "RHV"
  [FrontScrew] -> Add26/1
  [RearScrew] -> Add27/1
  [FRH] -> Subtract12/1
  [RRH] -> Subtract12/2
  Constant33/1 -> Atan2/2
  Subtract12/1 -> Atan2/1
  Atan2/1 -> Scope5/2, Add30/2  "Static Rake"
  [sigma] -> Scope5/1, Add30/1  "Dynamic Rake"
  Add30/1 -> Scope5/3, Gain57/1  "Total Rake"
  Gain57/1 -> [Rake]
  Integrator3/1 -> Scope13/1, [sigma]  "sigma"
  [FRH] -> Scope40/3  "FRH"
  Rear Suspension/5(M_Rear_R) -> [M_Rear_R]
  [z_w_R_L_dot] -> Rear Suspension/3(Z_w_R_L_dot)
  Front Suspension/2(F_Front_L) -> Scope9/1, [F_Front_L]
  [z_w_R_L] -> Rear Suspension/2(z_w_R_L)  "z_w_r"
  Rear Suspension/1(M_roll_Rear) -> [M_Roll_Rear]
  [z_w_F_R] -> Front Suspension/4(z_w_F_R)  "z_w_f"
  [z_w_F_L] -> Front Suspension/2(z_w_F_L)  "z_w_f"
  [z_w_F_L_dot] -> Front Suspension/3(Z_w_F_L_dot)
  Rear Suspension/2(F_Rear_L) -> [F_Rear_L], Scope9/3
  Front Suspension/4(F_Front_R) -> [F_Front_R]
  [theta_w_F] -> Front Suspension/1(sigma)
  [theta_w_R_dot] -> Rear Suspension/6(sigma_dot)
  [z_w_R_R] -> Rear Suspension/4(z_w_R_R)  "z_w_r"
  [z_w_F_R_dot] -> Front Suspension/5(Z_w_F_R_dot)
  [theta_w_R] -> Rear Suspension/1(sigma)
  Front Suspension/3(M_Front_L) -> Scope9/2, [M_Front_L]
  Front Suspension/5(M_Front_R) -> [M_Front_R]
  Rear Suspension/3(M_Rear_L) -> [M_Rear_L]
  [theta_w_F_dot] -> Front Suspension/6(sigma_dot)
  [z_w_R_R_dot] -> Rear Suspension/5(Z_w_R_R_dot)
  Front Suspension/1(M_roll_Front) -> [M_Roll_Front]
  Rear Suspension/4(F_Rear_R) -> Scope9/4, [F_Rear_R]
  Subtract14/1 -> Gain64/1
  Add25/1 -> [theta_w_F_dot]
  [z_us_FR_dot] -> Subtract13/2
  [z_us_RL_dot] -> Subtract14/1
  Subtract13/1 -> Gain62/1
  [z_us_FL_dot] -> Subtract13/1
  Gain64/1 -> Add29/2
  [theta_dot] -> Add29/1
  Gain62/1 -> Add25/2
  Add29/1 -> [theta_w_R_dot]
  [theta_dot] -> Add25/1
  [z_us_RR_dot] -> Subtract14/2
  Integrator4/1 -> Integrator5/1, [theta_dot]  "theta_dot"
  ay/1 -> Scope7/1, Scope1/1, Gain8/1, Gain4/1, Gain2/1, Divide1/1, Gain/1  "ay"
  Constant15/1 -> Add26/4
  Constant34/1 -> Add27/4
  Constant35/1 -> Add27/3
  Constant39/1 -> Add26/3
  [FrontScrew] -> Mux3/1  "FrontScrew"
  [RearScrew] -> Mux3/2  "RearScrew"
  Mux3/1 -> Scope41/2
  [vx] -> Scope41/1
  MATLAB Function/1(Delay) -> Time Delay/2
  vx/1 -> MATLAB Function/1(vx), [vx]
  z_t_R_L1/1 -> Mux4/4  "road_RL"
  Time Delay/1 -> Demux1/1
  Demux1/1 -> [z_t_FR]
  Demux1/4 -> [z_t_RL]
  z_t_F_L1/1 -> Mux4/2  "road_FL"
  z_t_F_R1/1 -> Scope7/2, Mux4/1  "road_FR"
  z_t_R_R1/1 -> Mux4/3  "road_RR"
  Demux1/2 -> [z_t_FL]
  Demux1/3 -> [z_t_RR]
  Mux4/1 -> Time Delay/1
  Actuator Dynamics1/1(ActuatorAccel) -> Actuator Performance Limits1/1(ActuatorAccel)
  Actuator Performance Limits1/2(Rear Actuators) -> Mux5/2, [RearScrew]  "Rear Position"
  Screw jack Reference - Road Conditions1/2(Screwjack_Reference_R) -> Mux6/2
  Screw jack Reference - Car Velocity1/2(Pitch_Reference_R) -> Mux7/2
  Sum23/1 -> Scope44/1, Controller1/1(Reference States)  "Position Reference"
  Screw jack Reference - Road Conditions1/1(Screwjack_Reference_F) -> Mux6/1
  Mux5/1 -> Scope44/2, Controller1/2(Current States)  "Output"
  [vx] -> Scope8/1, Transfer Fcn2/1
  Abs1/1 -> Transfer Fcn1/1
  [z_t_FR] -> Abs1/1
  Transfer Fcn1/1 -> Scope22/1, Screw jack Reference - Road Conditions1/1(Road_Input)
  Mux6/1 -> Scope22/2, Sum23/1
  Controller1/1(ActuatorTorque_cmd) -> Actuator Dynamics1/1(ActuatorTorque_cmd)
  Screw jack Reference - Car Velocity1/1(Pitch_Reference_F) -> Mux7/1
  Actuator Performance Limits1/1(Front Actuators) -> Mux5/1, [FrontScrew]  "Front Position"
  Mux7/1 -> Sum23/2, Scope16/3
  [CR] -> Scope16/2, Screw jack Reference - Car Velocity1/2(CR)
  Transfer Fcn2/1 -> Scope8/2, Scope16/1, Screw jack Reference - Car Velocity1/1(vx)
  MATLAB Function5/1(y) -> Scope15/1  "Ft_FR_Hist"
  [F_Front_L] -> MATLAB Function6/1(u), Sum10/1
  MATLAB Function6/1(y) -> Scope45/1  "Ft_FL_Hist"
  [F_Rear_R] -> MATLAB Function7/1(u), Sum11/1
  MATLAB Function7/1(y) -> Scope46/1  "Ft_RR_Hist"
  [F_Rear_L] -> MATLAB Function8/1(u), Sum14/1
  MATLAB Function8/1(y) -> Scope47/1  "Ft_RL_Hist"

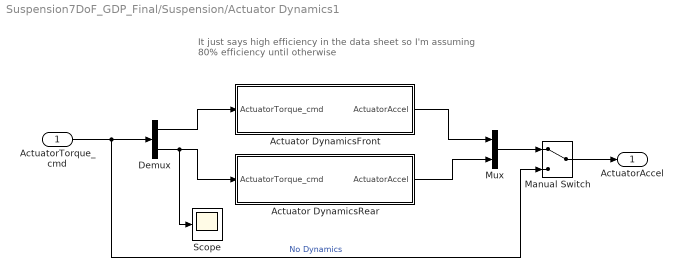
== system Suspension7DoF_GDP_Final/Suspension/Actuator Dynamics1 ==
  note: It just says high efficiency in the data sheet
      | so I'm assuming 80% efficiency until otherwise
  ActuatorTorque_cmd : Inport
  Actuator DynamicsFront : MATLAB Function  TreatAsAtomicUnit=on
  Actuator DynamicsRear : MATLAB Function  TreatAsAtomicUnit=on
  Demux : Demux  Outputs=2
  Manual Switch : ManualSwitch
  Mux : Mux  Inputs=2
  Scope : Scope
      settings: ActiveDisplayYMinimum=-0.0355999904028566  ActiveDisplayYMaximum=0.053400026711428517  DataLoggingVariableName=ScopeData21
  ActuatorAccel : Outport
  wires:
  Actuator DynamicsFront/1(ActuatorAccel) -> Mux/1
  ActuatorTorque_cmd/1 -> Manual Switch/2, Demux/1  "No Dynamics"
  Demux/1 -> Actuator DynamicsFront/1(ActuatorTorque_cmd)
  Demux/2 -> Scope/1, Actuator DynamicsRear/1(ActuatorTorque_cmd)
  Actuator DynamicsRear/1(ActuatorAccel) -> Mux/2
  Manual Switch/1 -> ActuatorAccel/1
  Mux/1 -> Manual Switch/1

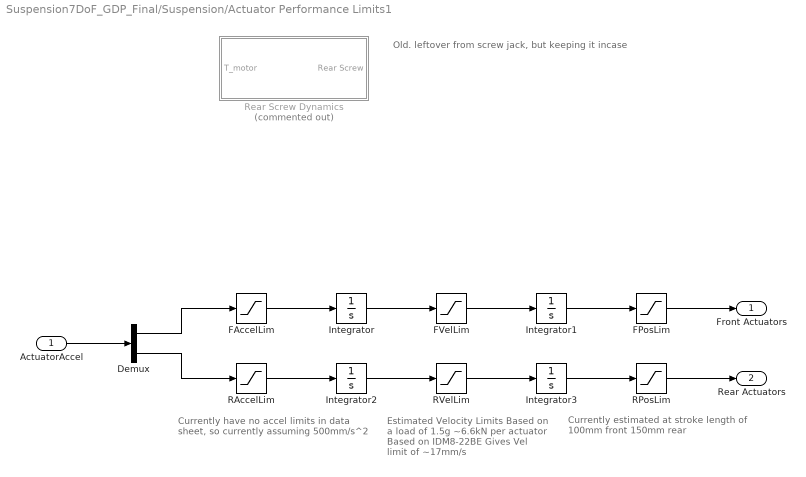
== system Suspension7DoF_GDP_Final/Suspension/Actuator Performance Limits1 ==
  note: Currently have no accel
      | limits in data sheet, so
      | currently assuming 500mm/s^2
  note: Currently estimated at
      | stroke length of 100mm front
      | 150mm rear
  note: Estimated Velocity Limits
      | Based on a load of 1.5g
      | ~6.6kN per actuator
      | Based on IDM8-22BE
      | Gives Vel limit of ~17mm/s
  note: Old. leftover from screw jack, but keeping it incase
  ActuatorAccel : Inport
  Demux : Demux  Outputs=2
  FAccelLim : Saturate  UpperLimit=1  LowerLimit=-1
  FPosLim : Saturate  UpperLimit=0.1  LowerLimit=0
  FVelLim : Saturate  UpperLimit=0.035  LowerLimit=-0.035
  Integrator{,1..3} (4 alike) : Integrator
  RAccelLim : Saturate  UpperLimit=1  LowerLimit=-1
  RPosLim : Saturate  UpperLimit=0.15  LowerLimit=0
  RVelLim : Saturate  UpperLimit=0.035  LowerLimit=-0.035
  Rear Screw Dynamics : Subsystem  Commented=on
  Front Actuators : Outport
  Rear Actuators : Outport  Port=2
  wires:
  ActuatorAccel/1 -> Demux/1
  Demux/1 -> FAccelLim/1
  Integrator1/1 -> FPosLim/1
  FAccelLim/1 -> Integrator/1
  FVelLim/1 -> Integrator1/1
  FPosLim/1 -> Front Actuators/1
  RVelLim/1 -> Integrator3/1
  RAccelLim/1 -> Integrator2/1
  Integrator3/1 -> RPosLim/1
  RPosLim/1 -> Rear Actuators/1
  Demux/2 -> RAccelLim/1
  Integrator/1 -> FVelLim/1
  Integrator2/1 -> RVelLim/1

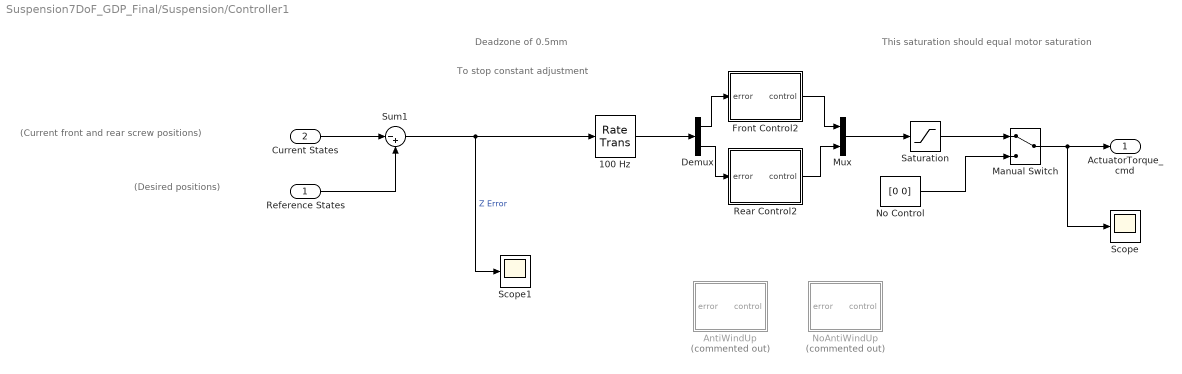
== system Suspension7DoF_GDP_Final/Suspension/Controller1 ==
  note: Deadzone of 0.5mm
  note: To stop constant adjustment
  note: This saturation should equal motor saturation
  note: (Desired positions)
  note: (Current front and rear screw positions)
  Reference States : Inport
  Current States : Inport  Port=2
  100 Hz : RateTransition  OutPortSampleTime=0.01
  AntiWindUp : MATLAB Function  Commented=on  TreatAsAtomicUnit=on
  Demux : Demux  Outputs=2
  Front Control2 : MATLAB Function  TreatAsAtomicUnit=on
  Manual Switch : ManualSwitch
  Mux : Mux  Inputs=2
  No Control : Constant  Value=[0 0]
  NoAntiWindUp : MATLAB Function  Commented=on  TreatAsAtomicUnit=on
  Rear Control2 : MATLAB Function  TreatAsAtomicUnit=on
  Saturation : Saturate  UpperLimit=14000  LowerLimit=-14000
  Scope : Scope
      settings: Title=Commanded Torque  ActiveDisplayYMinimum=-0.46538112917514463  ActiveDisplayYMaximum=0.73382043657501594  DataLoggingVariableName=ScopeData8
  Scope1 : Scope
      settings: ActiveDisplayYMinimum=-1  ActiveDisplayYMaximum=1  DataLoggingVariableName=ScopeData12
  Sum1 : Sum  Inputs=|-+
  ActuatorTorque_cmd : Outport
  wires:
  Manual Switch/1 -> Scope/1, ActuatorTorque_cmd/1
  Current States/1 -> Sum1/1
  No Control/1 -> Manual Switch/2
  Sum1/1 -> 100 Hz/1, Scope1/1  "Z Error"
  Saturation/1 -> Manual Switch/1
  Reference States/1 -> Sum1/2
  Mux/1 -> Saturation/1
  Rear Control2/1(control) -> Mux/2
  Demux/2 -> Rear Control2/1(error)
  Demux/1 -> Front Control2/1(error)
  Front Control2/1(control) -> Mux/1
  100 Hz/1 -> Demux/1

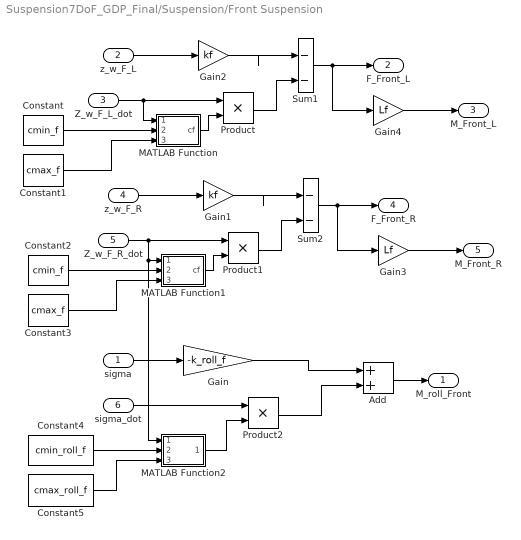
== system Suspension7DoF_GDP_Final/Suspension/Front Suspension ==
  sigma : Inport
  z_w_F_L : Inport  Port=2
  Z_w_F_L_dot : Inport  Port=3
  z_w_F_R : Inport  Port=4
  Z_w_F_R_dot : Inport  Port=5
  sigma_dot : Inport  Port=6
  Add : Sum
  Constant : Constant  Value=cmin_f
  Constant1 : Constant  Value=cmax_f
  Constant2 : Constant  Value=cmin_f
  Constant3 : Constant  Value=cmax_f
  Constant4 : Constant  Value=cmin_roll_f
  Constant5 : Constant  Value=cmax_roll_f
  Gain : Gain  Gain=-k_roll_f
  Gain1 : Gain  Gain=kf
  Gain2 : Gain  Gain=kf
  Gain3 : Gain  Gain=Lf
  Gain4 : Gain  Gain=Lf
  MATLAB Function : MATLAB Function  TreatAsAtomicUnit=on
  MATLAB Function1 : MATLAB Function  TreatAsAtomicUnit=on
  MATLAB Function2 : MATLAB Function  TreatAsAtomicUnit=on
  Product : Product
  Product1 : Product
  Product2 : Product
  Sum1 : Sum  Inputs=|--
  Sum2 : Sum  Inputs=|--
  M_roll_Front : Outport
  F_Front_L : Outport  Port=2
  M_Front_L : Outport  Port=3
  F_Front_R : Outport  Port=4
  M_Front_R : Outport  Port=5
  wires:
  sigma/1 -> Gain/1
  Gain2/1 -> Sum1/1
  Product/1 -> Sum1/2
  z_w_F_L/1 -> Gain2/1
  Z_w_F_L_dot/1 -> Product/1, MATLAB Function/1(z_w_f_dot)
  Sum1/1 -> Gain4/1, F_Front_L/1
  Gain4/1 -> M_Front_L/1
  MATLAB Function/1(cf) -> Product/2
  Constant/1 -> MATLAB Function/2(cmin_f)
  Constant1/1 -> MATLAB Function/3(cmax_f)
  z_w_F_R/1 -> Gain1/1
  Constant2/1 -> MATLAB Function1/2(cmin_f)
  Product1/1 -> Sum2/2
  Gain3/1 -> M_Front_R/1
  MATLAB Function1/1(cf) -> Product1/2
  Sum2/1 -> Gain3/1, F_Front_R/1
  Gain1/1 -> Sum2/1
  Z_w_F_R_dot/1 -> Product1/1, MATLAB Function2/1(z_w_f_dot), MATLAB Function1/1(z_w_f_dot)
  Constant3/1 -> MATLAB Function1/3(cmax_f)
  Add/1 -> M_roll_Front/1
  Gain/1 -> Add/1
  sigma_dot/1 -> Product2/1
  Constant4/1 -> MATLAB Function2/2(c_roll_min_f)
  Constant5/1 -> MATLAB Function2/3(c_roll_max_f)
  MATLAB Function2/1(c_roll_f) -> Product2/2
  Product2/1 -> Add/2

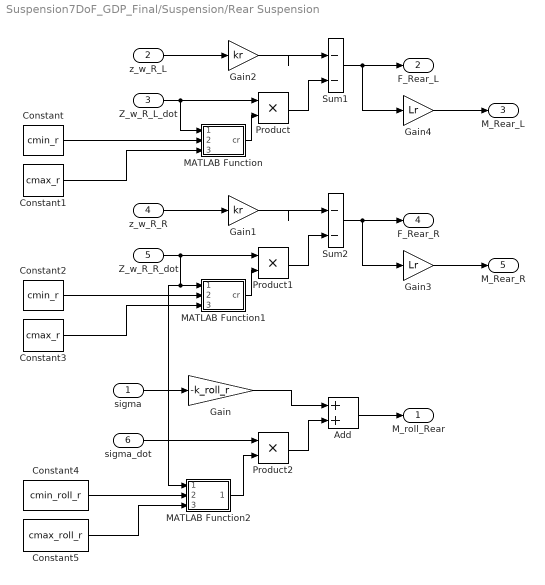
== system Suspension7DoF_GDP_Final/Suspension/Rear Suspension ==
  sigma : Inport
  z_w_R_L : Inport  Port=2
  Z_w_R_L_dot : Inport  Port=3
  z_w_R_R : Inport  Port=4
  Z_w_R_R_dot : Inport  Port=5
  sigma_dot : Inport  Port=6
  Add : Sum
  Constant : Constant  Value=cmin_r
  Constant1 : Constant  Value=cmax_r
  Constant2 : Constant  Value=cmin_r
  Constant3 : Constant  Value=cmax_r
  Constant4 : Constant  Value=cmin_roll_r
  Constant5 : Constant  Value=cmax_roll_r
  Gain : Gain  Gain=-k_roll_r
  Gain1 : Gain  Gain=kr
  Gain2 : Gain  Gain=kr
  Gain3 : Gain  Gain=Lr
  Gain4 : Gain  Gain=Lr
  MATLAB Function : MATLAB Function  TreatAsAtomicUnit=on
  MATLAB Function1 : MATLAB Function  TreatAsAtomicUnit=on
  MATLAB Function2 : MATLAB Function  TreatAsAtomicUnit=on
  Product : Product
  Product1 : Product
  Product2 : Product
  Sum1 : Sum  Inputs=|--
  Sum2 : Sum  Inputs=|--
  M_roll_Rear : Outport
  F_Rear_L : Outport  Port=2
  M_Rear_L : Outport  Port=3
  F_Rear_R : Outport  Port=4
  M_Rear_R : Outport  Port=5
  wires:
  Gain4/1 -> M_Rear_L/1
  sigma/1 -> Gain/1
  Product/1 -> Sum1/2
  Z_w_R_L_dot/1 -> Product/1, MATLAB Function/1(z_w_f_dot)
  Sum1/1 -> Gain4/1, F_Rear_L/1
  Gain2/1 -> Sum1/1
  z_w_R_L/1 -> Gain2/1
  MATLAB Function/1(cr) -> Product/2
  Constant/1 -> MATLAB Function/2(cmin_r)
  Constant1/1 -> MATLAB Function/3(cmax_r)
  Gain1/1 -> Sum2/1
  MATLAB Function1/1(cr) -> Product1/2
  Constant3/1 -> MATLAB Function1/3(cmax_r)
  Z_w_R_R_dot/1 -> Product1/1, MATLAB Function2/1(z_w_f_dot), MATLAB Function1/1(z_w_f_dot)
  Product1/1 -> Sum2/2
  Constant2/1 -> MATLAB Function1/2(cmin_r)
  Sum2/1 -> Gain3/1, F_Rear_R/1
  z_w_R_R/1 -> Gain1/1
  Gain3/1 -> M_Rear_R/1
  sigma_dot/1 -> Product2/1
  Gain/1 -> Add/1
  Add/1 -> M_roll_Rear/1
  Product2/1 -> Add/2
  MATLAB Function2/1(c_roll_r) -> Product2/2
  Constant4/1 -> MATLAB Function2/2(c_roll_min_r)
  Constant5/1 -> MATLAB Function2/3(c_roll_max_r)

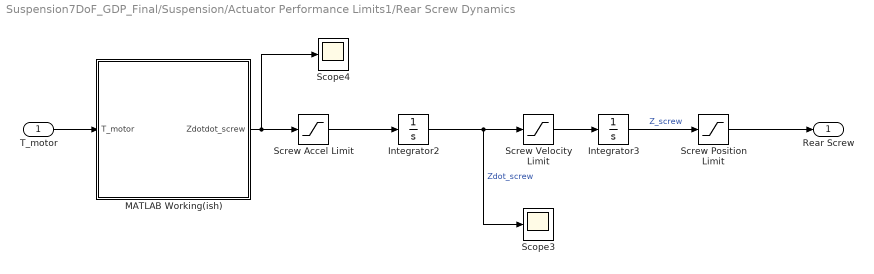
== system Suspension7DoF_GDP_Final/Suspension/Actuator Performance Limits1/Rear Screw Dynamics ==
  T_motor : Inport
  Integrator2 : Integrator
  Integrator3 : Integrator
  MATLAB Working(ish) : MATLAB Function  TreatAsAtomicUnit=on
  Scope3 : Scope
      settings: ActiveDisplayYMinimum=-1  ActiveDisplayYMaximum=1  DataLoggingVariableName=ScopeData15
  Scope4 : Scope
      settings: ActiveDisplayYMinimum=-110.01481996316281  ActiveDisplayYMaximum=105.02430114902371  DataLoggingVariableName=ScopeData16
  Screw Accel Limit : Saturate  UpperLimit=2  LowerLimit=-2
  Screw Position Limit : Saturate  UpperLimit=0.1  LowerLimit=0
  Screw Velocity Limit : Saturate
  Rear Screw : Outport
  wires:
  T_motor/1 -> MATLAB Working(ish)/1(T_motor)
  Integrator2/1 -> Scope3/1, Screw Velocity Limit/1  "Zdot_screw"
  MATLAB Working(ish)/1(Zdotdot_screw) -> Scope4/1, Screw Accel Limit/1
  Screw Velocity Limit/1 -> Integrator3/1
  Screw Position Limit/1 -> Rear Screw/1
  Screw Accel Limit/1 -> Integrator2/1
  Integrator3/1 -> Screw Position Limit/1  "Z_screw"

== matlab function Suspension7DoF_GDP_Final/Suspension/MATLAB Function8 ==
  data: u input; y output
function y = fcn(u)

if u > 0 
    y = u;
else
    y = 0;
end
end

== matlab function Suspension7DoF_GDP_Final/Suspension/Actuator Dynamics1/Actuator DynamicsFront ==
  data: ActuatorTorque_cmd input; ActuatorAccel output
function ActuatorAccel = fcn(ActuatorTorque_cmd)

%% Parameters

eta = 0.8; % Efficiency
L = 0.005; % Lead of Screw (m/rev)
Mass = 1775; % Mass of Car
M_a = 0.4491 * Mass; % Mass on Front Axle

ActuatorForce = (2*pi*eta*ActuatorTorque_cmd/L);

ActuatorAccel = 2*ActuatorForce/M_a;

end

== matlab function Suspension7DoF_GDP_Final/Suspension/Actuator Dynamics1/Actuator DynamicsRear ==
  data: ActuatorTorque_cmd input; ActuatorAccel output
function ActuatorAccel = fcn(ActuatorTorque_cmd)

%% Parameters

eta = 0.8; % Efficiency
L = 0.005; % Lead of Screw (m/rev)
Mass = 1775; % Mass of Car
M_b = 0.5501 * Mass; % Mass on Front Axle

ActuatorForce = (2*pi*eta*ActuatorTorque_cmd/L);

ActuatorAccel = 2*ActuatorForce/M_b;

end

== matlab function Suspension7DoF_GDP_Final/Suspension/Rear Suspension/MATLAB Function1 ==
  data: z_w_f_dot input; cr output; cmin_r input; cmax_r input
function cr = fcn(z_w_f_dot, cmin_r, cmax_r)

if abs(z_w_f_dot) > 0.1
    cr = cmin_r;
else 
    cr = cmax_r;
end

== matlab function Suspension7DoF_GDP_Final/Suspension/Rear Suspension/MATLAB Function2 ==
  data: z_w_f_dot input; c_roll_r output; c_roll_min_r input; c_roll_max_r input
function c_roll_r = fcn(z_w_f_dot, c_roll_min_r, c_roll_max_r)

if abs(z_w_f_dot) > 0.1
    c_roll_r = -c_roll_min_r;
else 
    c_roll_r = -c_roll_max_r;
end

== matlab function Suspension7DoF_GDP_Final/Suspension/MATLAB Function ==
  data: vx input; Delay output
function Delay = fcn(vx)

if vx > 5
    D = 25; % metres. Look ahead distance for Marie's road profile camer    
    Delay = D / vx;
else 
    Delay = 0;
end

== matlab function Suspension7DoF_GDP_Final/Suspension/Actuator Performance Limits1/Rear Screw Dynamics/MATLAB Working(ish) ==
  data: T_motor input; Zdotdot_screw output
function Zdotdot_screw  = Screw_Jack(T_motor)

L = 0.0005;        % lead (m/rev)
eta = 0.3;        % efficiency
Mass = 1754; % Car Mass (kg)
M_b = 0.5501 * Mass; % Mass on Rear axle (kg)
Friction = 150; % Screw Friction (N)

Fgravity = 0.25 * M_b * 9.81;

% Torque -> Force conversion
F_motor = (2*pi*eta * T_motor/ L) ;

F_net = F_motor - Friction * sign(T_motor);

% Dynamics
Zdotdot_screw = (F_motor)/ Mass;

end

== matlab function Suspension7DoF_GDP_Final/Suspension/MATLAB Function1 ==
  data: u input; y output
function y = fcn(u)

if u > 0 
    y = u;
else
    y = 0;
end
end

== matlab function Suspension7DoF_GDP_Final/Suspension/Controller1/AntiWindUp ==
  data: error input; control output
function control = fcn(error)

persistent error_prev error_sum
if isempty(error_prev), error_prev = 0; error_sum = 0; 
end

Ts = 0.01; % Sampling Time

Ku = 0.565; % Ultimate Gain
Tu = 2.97; % Oscillation Period
Kp = 0.33 * Ku; % System Response Speed
Ki = 0.05 * Ku / Tu; % Eliminates Steady State Error
Kd = 0.03 * Ku * Tu; % Reduces overshoot and ocsillations

% Derivative
de = (error - error_prev) / Ts;

control_unsat = Kp * error + Ki * error_sum + Kd * de;

%Saturation
control = max(min(control_unsat, 2000), -2000);

if (control == control_unsat) || ...
   (control == 2000 && error < 0) || ...
   (control == -2000 && error > 0)

    error_sum = error_sum + error * Ts;
end

error_prev = error;

== matlab function Suspension7DoF_GDP_Final/Suspension/Controller1/Front Control2 ==
  data: error input; control output
function control = fcn(error)
persistent error_prev error_sum de_filt

if isempty(error_prev)
    error_prev = 0;
    error_sum  = 0;
    de_filt    = 0;
end

Ts = 0.01;

% Gains
Kp = 0.2;    % reduced further to kill oscillation % System Response Speed
Ki = 0.0005;    % slow integrator % Eliminates Steady State Error
Kd = 1.75;    % significantly increased derivative damping % Reduces overshoot and ocsillations

% Filtered derivative - higher N = less filtering, more derivative action
% Lower N = smoother but slower derivative response
N  = 5;        % reduced from 10 for smoother derivative
de_filt = (1 - N*Ts) * de_filt + N * (error - error_prev);
de = de_filt;

% Compute unsaturated output first for anti-windup check
control_unsat = Kp * error + Ki * error_sum + Kd * de;

% Anti-windup: freeze integrator when saturated
if abs(control_unsat) < 2000
    error_sum = error_sum + error * Ts;
end

% Hard reset integrator if error is very large (prevents windup on big steps)
if abs(error) > 0.3
    error_sum = 0;
end

control = Kp * error + Ki * error_sum + Kd * de;
control = max(min(control, 10000), -10000);

error_prev = error;

== matlab function Suspension7DoF_GDP_Final/Suspension/Controller1/NoAntiWindUp ==
  data: error input; control output
function control = fcn(error)

persistent error_prev error_sum
if isempty(error_prev), error_prev = 0; error_sum = 0; 
end

Ts = 0.2; % Sampling Time

Ku = 1; % Ultimate Gain
Tu = 5; % Oscillation Period
Kp = 0.02 * Ku; % System Response Speed
Ki = 0.0001 * Ku / Tu; % Eliminates Steady State Error
Kd = 0.35 * Ku * Tu; % Reduces overshoot and ocsillations

% PID Terms
error_sum = error_sum + error * Ts;
de = (error - error_prev) / Ts;

control = Kp * error + Ki * error_sum + Kd * de;

%Saturation
control = max(min(control, 2000), -2000);

error_prev = error;

== matlab function Suspension7DoF_GDP_Final/Suspension/Controller1/Rear Control2 ==
  data: error input; control output
function control = fcn(error)
persistent error_prev error_sum de_filt

if isempty(error_prev)
    error_prev = 0;
    error_sum  = 0;
    de_filt    = 0;
end

Ts = 0.01;

% Gains
Kp = 0.15;    % reduced further to kill oscillation % System Response Speed
Ki = 0.0005;    % slow integrator % Eliminates Steady State Error
Kd = 1.75;    % significantly increased derivative damping % Reduces overshoot and ocsillations

% Filtered derivative - higher N = less filtering, more derivative action
% Lower N = smoother but slower derivative response
N  = 5;        % reduced from 10 for smoother derivative
de_filt = (1 - N*Ts) * de_filt + N * (error - error_prev);
de = de_filt;

% Compute unsaturated output first for anti-windup check
control_unsat = Kp * error + Ki * error_sum + Kd * de;

% Anti-windup: freeze integrator when saturated
if abs(control_unsat) < 2000
    error_sum = error_sum + error * Ts;
end

% Hard reset integrator if error is very large (prevents windup on big steps)
if abs(error) > 0.3
    error_sum = 0;
end

control = Kp * error + Ki * error_sum + Kd * de;
control = max(min(control, 10000), -10000);

error_prev = error;

== matlab function Suspension7DoF_GDP_Final/Suspension/Screw jack Reference - Car Velocity1 ==
  data: vx input; Pitch_Reference_F output; Pitch_Reference_R output; CR input
function [Pitch_Reference_F, Pitch_Reference_R] = fcn(vx,CR)

% Predefined Ride Heights at certain velocities - minimise rake at high
% speed, maximise effective rake at low speed
Low_Speed = [0 0.0]; 
Med_Speed = [0 0.05]; % Should be 1.5 degrees
High_Speed = [0 0.1]; % Should be >2 degrees

% Thresholds in ascending order
Thresholds = [20, 30]; % ms^-1

% Corresponding Ride Heights
Ride_Heights = [Low_Speed, Med_Speed, High_Speed];

Pitch_Reference_F = 0;
Pitch_Reference_R = 0;

if abs(CR) < 500  % Only adjust pitch in corners
    Pitch_Reference_F = Ride_Heights(end-1);
    Pitch_Reference_R = Ride_Heights(end);
    for i = 1:length(Thresholds)
        if vx < Thresholds(i)
            Pitch_Reference_F = Ride_Heights(2*i-1);
            Pitch_Reference_R = Ride_Heights(2*i);
            return;
        end
    end
end
end

== matlab function Suspension7DoF_GDP_Final/Suspension/Screw jack Reference - Road Conditions1 ==
  data: Road_Input input; Screwjack_Reference_F output; Screwjack_Reference_R output
function [Screwjack_Reference_F,Screwjack_Reference_R]  = fcn(Road_Input)

% Predefined Ride Heights - Can add pitch by adjusting reference states
Tarmac = [0 0];
Gravel = [0.075 0.075];

% Thresholds in ascending order
Height_Thresholds = 0.02;

% Corresponding Ride Heights
Ride_Heights = [Tarmac, Gravel];

Screwjack_Reference_F = Ride_Heights(end-1);
Screwjack_Reference_R = Ride_Heights(end);

for i = 1:length(Height_Thresholds)
    if Road_Input < Height_Thresholds(i)
        Screwjack_Reference_F = Ride_Heights(2*i-1);
        Screwjack_Reference_R = Ride_Heights(2*i);
        return;
    end
end

end

== matlab function Suspension7DoF_GDP_Final/Suspension/MATLAB Function4 ==
  data: u input; y output
function y = fcn(u)

if u > 0 
    y = u;
else
    y = 0;
end
end

== matlab function Suspension7DoF_GDP_Final/Suspension/MATLAB Function2 ==
  data: u input; y output
function y = fcn(u)

if u > 0 
    y = u;
else
    y = 0;
end
end

== matlab function Suspension7DoF_GDP_Final/Suspension/MATLAB Function3 ==
  data: u input; y output
function y = fcn(u)

if u > 0 
    y = u;
else
    y = 0;
end
end

== matlab function Suspension7DoF_GDP_Final/Suspension/Front Suspension/MATLAB Function ==
  data: z_w_f_dot input; cf output; cmin_f input; cmax_f input
function cf = fcn(z_w_f_dot, cmin_f, cmax_f)

if abs(z_w_f_dot) > 0.1
    cf = cmin_f;
else 
    cf = cmax_f;
end

== matlab function Suspension7DoF_GDP_Final/Suspension/Front Suspension/MATLAB Function2 ==
  data: z_w_f_dot input; c_roll_f output; c_roll_min_f input; c_roll_max_f input
function c_roll_f = fcn(z_w_f_dot, c_roll_min_f, c_roll_max_f)

if abs(z_w_f_dot) > 0.1
    c_roll_f = -c_roll_min_f;
else 
    c_roll_f = -c_roll_max_f;
end

== matlab function Suspension7DoF_GDP_Final/Suspension/Front Suspension/MATLAB Function1 ==
  data: z_w_f_dot input; cf output; cmin_f input; cmax_f input
function cf = fcn(z_w_f_dot, cmin_f, cmax_f)

if abs(z_w_f_dot) > 0.1
    cf = cmin_f;
else 
    cf = cmax_f;
end

== matlab function Suspension7DoF_GDP_Final/Suspension/Rear Suspension/MATLAB Function ==
  data: z_w_f_dot input; cr output; cmin_r input; cmax_r input
function cr = fcn(z_w_f_dot, cmin_r, cmax_r)

if abs(z_w_f_dot) > 0.1
    cr = cmin_r;
else 
    cr = cmax_r;
end

== matlab function Suspension7DoF_GDP_Final/Suspension/MATLAB Function5 ==
  data: u input; y output
function y = fcn(u)

if u > 0 
    y = u;
else
    y = 0;
end
end

== matlab function Suspension7DoF_GDP_Final/Suspension/MATLAB Function6 ==
  data: u input; y output
function y = fcn(u)

if u > 0 
    y = u;
else
    y = 0;
end
end

== matlab function Suspension7DoF_GDP_Final/Suspension/MATLAB Function7 ==
  data: u input; y output
function y = fcn(u)

if u > 0 
    y = u;
else
    y = 0;
end
end
